simulink model "Self_phase_inductor_with_RL_load"  (R2013a)
settings: Solver=ode45  StartTime=0.0  StopTime=10.0  RelTol=1e-3
libraries: powerlib x9, powerlib_meascontrol x2
settings Model: Creator=user  LastModifiedBy=user

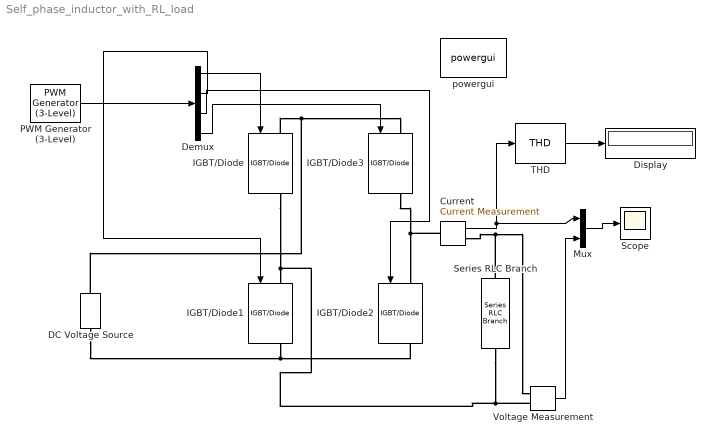
== system Self_phase_inductor_with_RL_load ==
  "Current " : powerlib/Measurements/Current Measurement  PhasorSimulation=off  OutputType=Complex  PSBequivalent=0
  DC Voltage Source : powerlib/Electrical Sources/DC Voltage Source  Amplitude=100  Measurements=None
  Demux : Demux
  Display : Display
  IGBT/Diode{,1..3} (4 alike) : powerlib/Power Electronics/IGBT//Diode  Ron=1e-3  Rs=1e5  Cs=inf  Measurements=on
  Mux : Mux  Inputs=2
  PWM Generator (3-Level) : powerlib_meascontrol/Pulse & Signal Generators/PWM Generator (3-Level)  ModulatorType=Single-phase half-bridge (4 pulses)  ModulatorMode=Unsynchronized  nF=27  Fc=1080  ModulatingSignals=on  m=0.8  Freq=50  Phase=0  Ts=0
  Scope : Scope
      settings: YMin=-4e-07  YMax=4e-07
  Series RLC Branch : powerlib/Elements/Series RLC Branch  LConnTagsString=__new0  RConnTagsString=__new0  BranchType=RL  Resistance=1  Inductance=1e-3  SetiL0=off  InitialCurrent=0  Capacitance=0  Setx0=off  InitialVoltage=0  Measurements=Branch voltage
  THD : powerlib_meascontrol/Measurements/THD  Freq=60  Ts=0
  Voltage Measurement : powerlib/Measurements/Voltage Measurement  PhasorSimulation=off  OutputType=Complex  PSBequivalent=0
  powergui : powerlib/powergui  Priority=1  SimulationMode=Discrete  SolverType=Tustin  SampleTime=50e-6  frequency=60  SPID=off  DisableSnubberDevices=off  DisableRonSwitches=off  DisableVfSwitches=off  SwTol=0  Interpol=off  DisplayEquations=off  frequencyindice=0  Pbase=100e6  ErrMax=1e-4  Iterations=50  UnitsV=kV  UnitsW=MW  FunctionMessages=off  echomessages=off  HookPort=off  EnableUseOfTLC=off  x0status=blocks  RestoreLinks=warning  ResistiveCurrentMeasurement=off  Frange=[0:2:500]  Ylog=off  Xlog=on  ShowGrid=off  save=off  variable=ZData  ZoomFFT=off  StartTime=0.0  cycles=1  DisplayStyle=1  fundamental=60  FreqAxis=off  MaxFrequency=1000  frequencyindicesteady=1  RmsSteady=1  display=off  Ts=0  methode=off
  wires:
  PWM Generator (3-Level)/1 -> Demux/1
  Demux/4 -> IGBT/Diode3/1
  Demux/3 -> IGBT/Diode2/1
  Demux/2 -> IGBT/Diode1/1
  Demux/1 -> IGBT/Diode/1
  "Current "/1 -> THD/1, Mux/1
  Voltage Measurement/1 -> Mux/2
  THD/1 -> Display/1
  Mux/1 -> Scope/1
  connections:
  IGBT/Diode/RConn1 -- Series RLC Branch/RConn1 -- Voltage Measurement/LConn2 -- IGBT/Diode1/LConn1
  IGBT/Diode3/RConn1 -- "Current "/LConn1 -- IGBT/Diode2/LConn1
  IGBT/Diode/LConn1 -- IGBT/Diode3/LConn1 -- DC Voltage Source/RConn1
  "Current "/RConn1 -- Series RLC Branch/LConn1 -- Voltage Measurement/LConn1
  IGBT/Diode1/RConn1 -- IGBT/Diode2/RConn1 -- DC Voltage Source/LConn1
